simulink model "Q2_Ball_Beam"  (R2018b)
settings: Solver=ode45  StartTime=0.0  StopTime=20  MaxStep=0.01  RelTol=1e-3  EnableMultiTasking=on
undefined symbols (not defined in the file): c, d, g, L, m, nG, nSat, nVR
libraries: slctrlblks x1, checkpacklib x1
settings Model: Creator=Home  LastModifiedBy=Erfan Etesami
settings DataIOCC: LimitDataPoints=on
settings OptimizationCC: LifeSpan=inf
settings DebuggingCC: SFUnexpectedBacktrackingDiag=warning  SFNoUnconditionalDefaultTransitionDiag=warning  SFExecutionAtInitializationDiag=none
settings HardwareCC: ProdBitPerSizeT=32  ProdBitPerPtrDiffT=32  ProdWordSize=32  ProdHWDeviceType=Specified
settings SFSimCC: SimUseLocalCustomCode=off
settings RTWCC: RTWUseLocalCustomCode=off
settings CodeAppCC: StateflowObjectComments=on
settings GRTTargetCC: TargetLangStandard=C89/C90 (ANSI)  GeneratePreprocessorConditionals=Disable all
settings ConfigComp: CovMetricSettings=dw  CovHtmlReporting=on  CovSaveCumulativeToWorkspaceVar=on  CovSaveSingleToWorkspaceVar=on  CovExternalEMLEnable=off  CovSFcnEnable=off
settings SimscapeCC: SimscapeNominalValues="[{\"value\":\"10\",\"unit\":\"V\"},{\"value\":\"1\",\"unit\":\"A\"},{\"value\":\"10\",\"unit\":\"N*m\"},{\"value\":\"10\",\"unit\":\"bar\"},{\"value\":\"100\",\"unit\":\"kJ/kg\"},{\"value\":\"1\",\"unit\":\"kW\"},{\"value\":\"300\",\"unit\":\"K\"},{\"value\":\"100\",\"unit\":\"cm^3/s\"},{\"value\":\"1\",\"unit\":\"kN\"},{\"value\":\"1\",\"unit\":\"g/cm^3\"},{\"value\":\"1\",\"unit\":\"l\"},{\"value\":\"1\",\"unit\":\"cm^2\"},{\"value\":\"60\",\"unit\":\"Hz\"}]"  SimscapeLogType=all  SimscapeLogDataHistory=10000

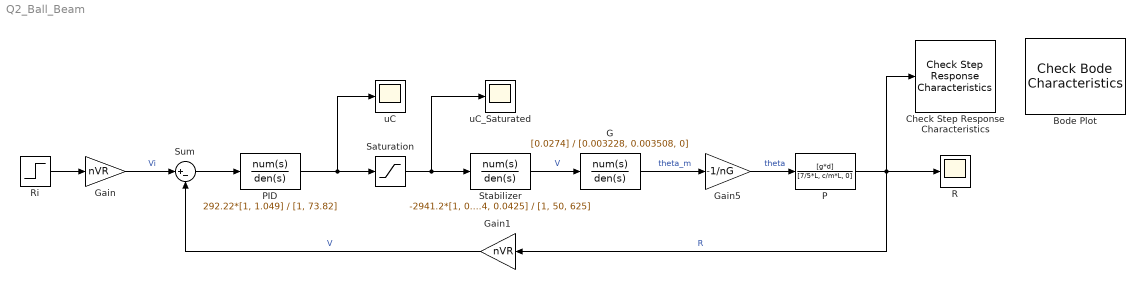
== system Q2_Ball_Beam ==
  " PID" : TransferFcn  Numerator=292.22*[1, 1.049]  Denominator=[1, 73.82]
  Bode Plot : slctrlblks/Model Verification/Check Bode  Characteristics  InstantiateOnLoad=on  SaveOperatingPoints=off  LinearizationIOs={'/P', 1, 'out', 'on', '';'/Ri ', 1, 'in', 'on', ''}  LinearizeAt=SnapshotTimes  SnapshotTimes=[0]  TriggerType=rising  SampleTime=auto  RateConversionMethod=zoh  PreWarpFreq=10  UseExactDelayModel=off  UseFullBlockNameLabels=off  UseBusSignalLabels=off  enabled=on  stopWhenAssertionFail=off  export=off  ViewDlgPos=[100 128.2 568.2 461.8]  OpenViewOnLoad=on  LaunchViewOnOpen=on  FrequencyUnits=rad/s  MagnitudeUnits=dB  PhaseUnits=deg  TimeUnits=seconds  EnableUpperBound=off  UpperBoundFrequencies=[]  UpperBoundMagnitudes=[]  EnableLowerBound=off  LowerBoundFrequencies=[]  LowerBoundMagnitudes=[]
      settings: SourceProductName=Simulink Control Design
  Check Step Response Characteristics : checkpacklib/Check Step Response  Characteristics  InstantiateOnLoad=on  enabled=on  stopWhenAssertionFail=on  export=off  ViewDlgPos=[241 204.2 509.6 389.6]  OpenViewOnLoad=off  LaunchViewOnOpen=on  TimeUnits=seconds  EnableStepResponseBound=on  InitialValue=0  FinalValue=L/2  StepTime=0  RiseTime=5  PercentRise=80  SettlingTime=6  PercentSettling=2  PercentOvershoot=20  PercentUndershoot=1
  G : TransferFcn  Numerator=[0.0274]  Denominator=[0.003228, 0.003508, 0]
  Gain : Gain  Gain=nVR
  Gain1 : Gain  Gain=nVR
  Gain5 : Gain  Gain=-1/nG
  P : TransferFcn  Numerator=[g*d]  Denominator=[7/5*L, c/m*L, 0]
  R : Scope
  "Ri " : Step  Time=0  After=L/2  SampleTime=0
  "Saturation " : Saturate  UpperLimit=nSat  LowerLimit=-nSat
  Stabilizer : TransferFcn  Numerator=-2941.2*[1, 0.4, 0.0425]  Denominator=[1, 50, 625]
  Sum : Sum  Inputs=|+-
  uC : Scope
  uC_Saturated : Scope
  wires:
  "Ri "/1 -> Gain/1
  Gain/1 -> Sum/1  "Vi"
  Sum/1 -> " PID"/1
  G/1 -> Gain5/1  "theta_m"
  Gain1/1 -> Sum/2  "V"
  P/1 -> Check Step Response Characteristics/1, R/1, Gain1/1  "R"
  Gain5/1 -> P/1  "theta"
  Stabilizer/1 -> G/1  "V"
  " PID"/1 -> "Saturation "/1, uC/1
  "Saturation "/1 -> Stabilizer/1, uC_Saturated/1
